simulink model "CDM_substructure"  (R2022b)
settings: Solver=FixedStepAuto  StartTime=0.0  StopTime=55.0  FixedStep=0.001  RelTol=1e-3
values from neighbouring files (symbols this model uses):
  a_ns = K_ns - (2 * M_ns) / (dt)^2    [Final_10DOFs_RTHS.m]    (also in ThreeDOFs_CDM_substructure.m; structure_2DOFs.m = -3998200)
  a_ps = K_ps - (2 * M_ps) / (dt)^2    (= -21398788.6)    [Final_10DOFs_RTHS.m]    (also in ThreeDOFs_CDM_substructure.m = -1999400; structure_2DOFs.m = -9.988)
  ACC_el = ACC_el(1:10000,:)    [ThreeDOFs_Dampling.m]    (also in ThreeDOFs_noDampling.m; multiDOFs_CDM_highspeed_Dampling.m = ACC_el(1:2000,:); multiDOFs_auto_for_loop.m = ACC_el(1:1000,:); multiDOFs_highspeed.m = ACC_el(1:1000,:))
  b_ns = M_ns / dt^2 - C_ns / (2*dt)    [Final_10DOFs_RTHS.m]    (also in ThreeDOFs_CDM_substructure.m; structure_2DOFs.m = 1850000)
  b_ps = M_ps / dt^2 - C_ps / (2*dt)    (= 10684932)    [Final_10DOFs_RTHS.m]    (also in ThreeDOFs_CDM_substructure.m = 924875; structure_2DOFs.m = 4)
  diagM_ns = diag(M_ns)    [Final_10DOFs_RTHS.m]    (also in ThreeDOFs_CDM_substructure.m; structure_2DOFs.m)
  dt = 0.001    [CDM_ACC_or_Disp_Input.m]    (also in Final_10DOFs_RTHS.m; ThreeDOFs_CDM_Dampling.m; ThreeDOFs_CDM_substructure.m; ThreeDOFs_Dampling.m)
  Ke_ns_inv = inv(Ke_ns)    [ThreeDOFs_CDM_substructure.m]
  Ke_ps_inv = inv(Ke_ps)    [Final_10DOFs_RTHS.m]    (also in ThreeDOFs_CDM_substructure.m)
  M_ps = m9 * 1e-5    (= 10.7)    [Final_10DOFs_RTHS.m]    (also in ThreeDOFs_CDM_substructure.m = 1; structure_2DOFs.m = 5e-06)
  ps_weizhi = zeros(length(M_ns),1)    [Final_10DOFs_RTHS.m]    (also in ThreeDOFs_CDM_substructure.m = [0 ; 1])
libraries: dspsrcs4 x2
settings Model: Creator=dongxh  LastModifiedBy=dongxh

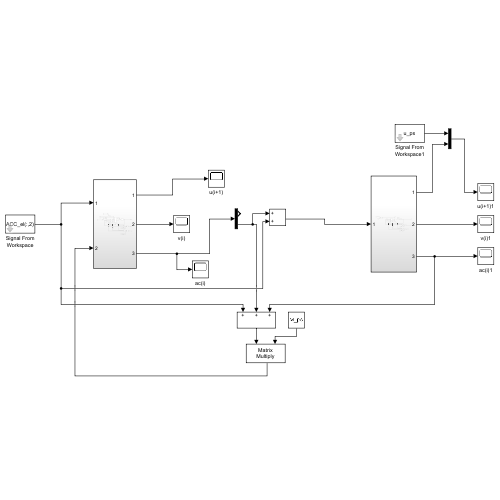
[thumbnail: Simulink's stored preview of the top-level diagram]
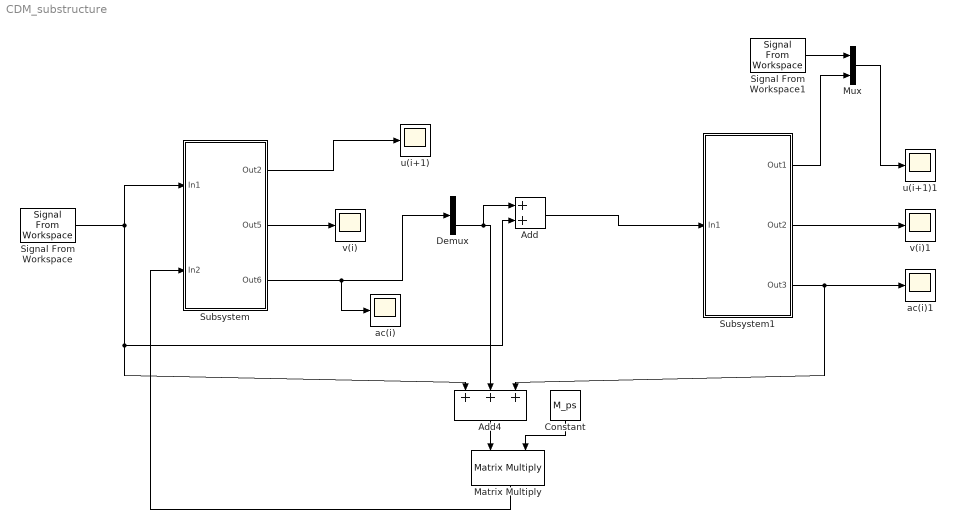
== system CDM_substructure ==
  Add : Sum
  Add4 : Sum  Inputs=+++
  Constant : Constant  Value=M_ps
  Demux : Demux  Outputs=2
  Matrix Multiply : Product  Multiplication=Matrix(*)
  Mux : Mux  Inputs=2
  Signal From Workspace : dspsrcs4/Signal From Workspace  X=ACC_el(:,2)  Ts=0.001  nsamps=1  OutputAfterFinalValue=Setting to zero  ignoreOrWarnInputAndFrameLengths=off  OutputFrames=off
  Signal From Workspace1 : dspsrcs4/Signal From Workspace  X=u_ps  Ts=0.001  nsamps=1  OutputAfterFinalValue=Setting to zero  ignoreOrWarnInputAndFrameLengths=off  OutputFrames=off
  Subsystem : Subsystem
  Subsystem1 : Subsystem
  ac(i) : Scope
  ac(i)1 : Scope
  u(i+1) : Scope
  u(i+1)1 : Scope
  v(i) : Scope
  v(i)1 : Scope
  wires:
  Signal From Workspace/1 -> Add/2, Add4/1, Subsystem/1(In1)
  Subsystem/2(Out5) -> v(i)/1
  Subsystem/3(Out6) -> ac(i)/1, Demux/1
  Demux/2 -> Add4/2, Add/1
  Subsystem1/3(Out3) -> Add4/3, ac(i)1/1
  Add/1 -> Subsystem1/1(In1)
  Subsystem1/2(Out2) -> v(i)1/1
  Add4/1 -> Matrix Multiply/1
  Constant/1 -> Matrix Multiply/2
  Matrix Multiply/1 -> Subsystem/2(In2)
  Subsystem1/1(Out1) -> Mux/2
  Mux/1 -> u(i+1)1/1
  Signal From Workspace1/1 -> Mux/1
  Subsystem/1(Out2) -> u(i+1)/1

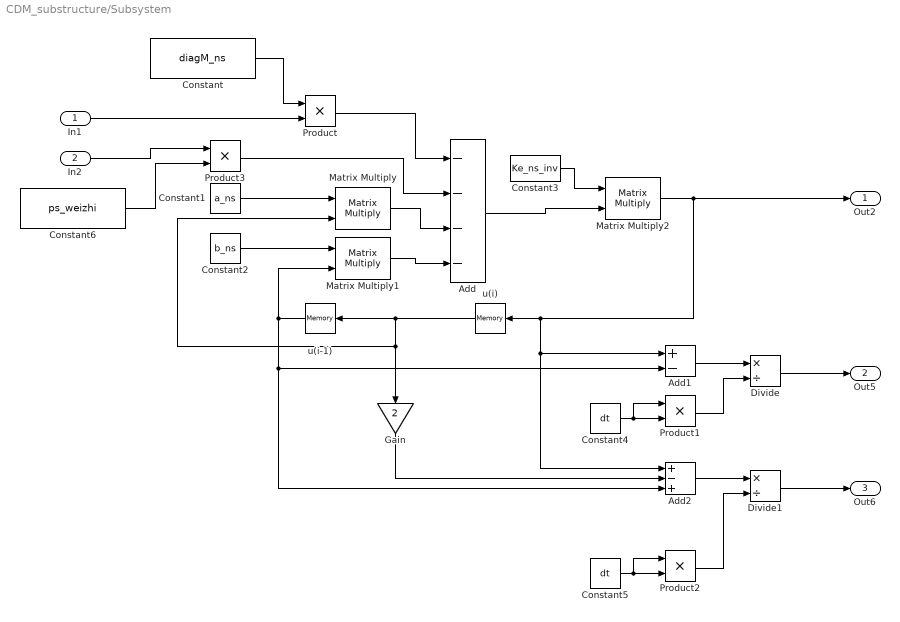
== system CDM_substructure/Subsystem ==
  In1 : Inport
  In2 : Inport  Port=2
  Add : Sum  Inputs=----
  Add1 : Sum  Inputs=+-
  Add2 : Sum  Inputs=+-+
  Constant : Constant  Value=diagM_ns  VectorParams1D=off
  Constant1 : Constant  Value=a_ns  VectorParams1D=off
  Constant2 : Constant  Value=b_ns  VectorParams1D=off
  Constant3 : Constant  Value=Ke_ns_inv  VectorParams1D=off
  Constant4 : Constant  Value=dt  VectorParams1D=off
  Constant5 : Constant  Value=dt  VectorParams1D=off
  Constant6 : Constant  Value=ps_weizhi  VectorParams1D=off
  Divide : Product  Inputs=*/
  Divide1 : Product  Inputs=*/
  Gain : Gain  Gain=2
  Matrix Multiply : Product  Multiplication=Matrix(*)
  Matrix Multiply1 : Product  Multiplication=Matrix(*)
  Matrix Multiply2 : Product  Multiplication=Matrix(*)
  Product{,1..3} (4 alike) : Product
  u(i) : Memory
  u(i-1) : Memory
  Out2 : Outport
  Out5 : Outport  Port=2
  Out6 : Outport  Port=3
  wires:
  u(i-1)/1 -> Matrix Multiply1/2, Add2/3, Add1/2
  u(i)/1 -> u(i-1)/1, Matrix Multiply/2, Gain/1
  Constant/1 -> Product/1
  Add/1 -> Matrix Multiply2/2
  Constant1/1 -> Matrix Multiply/1
  Add2/1 -> Divide1/1
  Product/1 -> Add/1
  Constant5/1 -> Product2/2, Product2/1
  Matrix Multiply2/1 -> Out2/1, Add2/1, Add1/1, u(i)/1
  Constant4/1 -> Product1/1, Product1/2
  Gain/1 -> Add2/2
  Product1/1 -> Divide/2
  Constant2/1 -> Matrix Multiply1/1
  Constant3/1 -> Matrix Multiply2/1
  Add1/1 -> Divide/1
  Divide1/1 -> Out6/1
  Product2/1 -> Divide1/2
  In1/1 -> Product/2
  Divide/1 -> Out5/1
  Matrix Multiply1/1 -> Add/4
  Matrix Multiply/1 -> Add/3
  Product3/1 -> Add/2
  In2/1 -> Product3/1
  Constant6/1 -> Product3/2

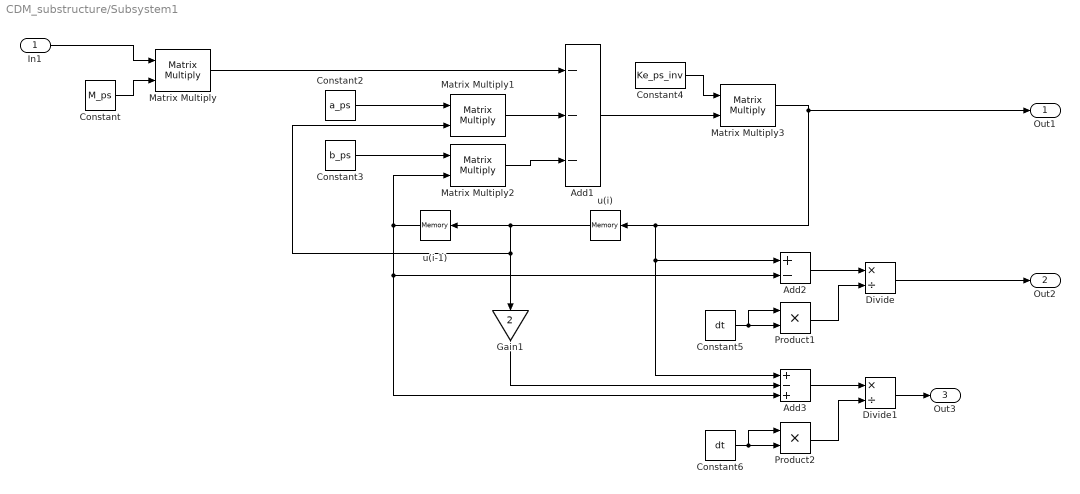
== system CDM_substructure/Subsystem1 ==
  In1 : Inport
  Add1 : Sum  Inputs=---
  Add2 : Sum  Inputs=+-
  Add3 : Sum  Inputs=+-+
  Constant : Constant  Value=M_ps
  Constant2 : Constant  Value=a_ps  VectorParams1D=off
  Constant3 : Constant  Value=b_ps  VectorParams1D=off
  Constant4 : Constant  Value=Ke_ps_inv  VectorParams1D=off
  Constant5 : Constant  Value=dt  VectorParams1D=off
  Constant6 : Constant  Value=dt  VectorParams1D=off
  Divide : Product  Inputs=*/
  Divide1 : Product  Inputs=*/
  Gain1 : Gain  Gain=2
  Matrix Multiply{,1..3} (4 alike) : Product  Multiplication=Matrix(*)
  Product1 : Product
  Product2 : Product
  u(i) : Memory
  u(i-1) : Memory
  Out1 : Outport
  Out2 : Outport  Port=2
  Out3 : Outport  Port=3
  wires:
  Matrix Multiply1/1 -> Add1/2
  Matrix Multiply/1 -> Add1/1
  Matrix Multiply3/1 -> Out1/1, Add3/1, Add2/1, u(i)/1
  Product2/1 -> Divide1/2
  Constant/1 -> Matrix Multiply/2
  u(i-1)/1 -> Matrix Multiply2/2, Add3/3, Add2/2
  Product1/1 -> Divide/2
  Constant3/1 -> Matrix Multiply2/1
  In1/1 -> Matrix Multiply/1
  u(i)/1 -> u(i-1)/1, Matrix Multiply1/2, Gain1/1
  Constant5/1 -> Product1/1, Product1/2
  Add2/1 -> Divide/1
  Constant4/1 -> Matrix Multiply3/1
  Constant6/1 -> Product2/2, Product2/1
  Constant2/1 -> Matrix Multiply1/1
  Gain1/1 -> Add3/2
  Add1/1 -> Matrix Multiply3/2
  Add3/1 -> Divide1/1
  Matrix Multiply2/1 -> Add1/3
  Divide1/1 -> Out3/1
  Divide/1 -> Out2/1
